simulink model "blank_canvas_ssc"  (R2025b)
settings: Solver=ode1  StartTime=0.0  StopTime=1  FixedStep=Ts  RelTol=1e-3  EnableMultiTasking=on
settings Model: SimulationMode=accelerator  Creator=gdudgeon  LastModifiedBy=gdudgeon
settings SolverCC: AlgebraicLoopSolver=TrustRegion  AutoInsertRateTranBlk=on
settings DataIOCC: ExternalInput=[t, load_inputs]  LoadExternalInput=on  SaveFormat=Array  SaveOutput=off  DSMLogging=off  InspectSignalLogs=on  VisualizeSimOutput=off  SaveTime=off
settings OptimizationCC: ExpressionDepthLimit=2147483647.0  LifeSpan=inf
settings DebuggingCC: UnderspecifiedInitializationDetection=Classic  MergeDetectMultiDrivingBlocksExec=none  SolverPrmCheckMsg=warning  UnconnectedInputMsg=warning  UnconnectedOutputMsg=warning  UnconnectedLineMsg=warning  StateNameClashWarn=warning  SFUnexpectedBacktrackingDiag=warning  SFNoUnconditionalDefaultTransitionDiag=warning  SFExecutionAtInitializationDiag=none  ArithmeticOperatorsInVariantConditions=warning
settings HardwareCC: ProdBitPerPointer=32.0  ProdBitPerSizeT=32.0  ProdBitPerPtrDiffT=32.0  ProdLargestAtomicFloat=None  ProdIntDivRoundTo=Undefined  ProdEndianess=Unspecified  ProdWordSize=32.0  ProdHWDeviceType=32-bit Generic
settings ModelReferenceCC: EnableRefExpFcnMdlSchedulingChecks=on  PropagateSignalLabelsOutOfModel=off
settings SFSimCC: SimUseLocalCustomCode=off  CustomCodeUndefinedFunction=UseInterfaceOnly
settings RTWCC: RTWUseLocalCustomCode=off  GPUComputeCapability=3.5
settings CodeAppCC: StateflowObjectComments=on
settings GRTTargetCC: TargetLangStandard=C89/C90 (ANSI)
settings ConfigComp: CovMetricSettings=dw  CovSaveCumulativeToWorkspaceVar=on  CovSaveSingleToWorkspaceVar=on  CovExternalEMLEnable=off  CovSFcnEnable=off
settings SimscapeCC: SimscapeNormalizeSystem=off
settings ConfigurationSet: Description=SimMechanics 2G

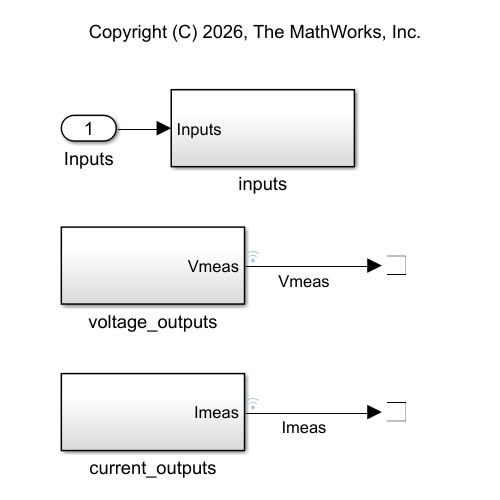
[thumbnail: Simulink's stored preview of the top-level diagram]
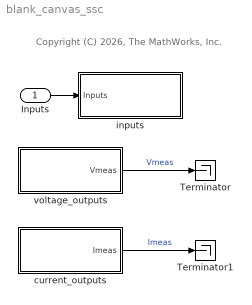
== system blank_canvas_ssc ==
  note: Copyright (C) 2026, The MathWorks, Inc.
  Inputs : Inport
  Terminator : Terminator
  Terminator1 : Terminator
  current_outputs : Subsystem
  inputs : Subsystem
  voltage_outputs : Subsystem
  wires:
  voltage_outputs/1(Vmeas) -> Terminator/1  "Vmeas"
  current_outputs/1(Imeas) -> Terminator1/1  "Imeas"
  Inputs/1 -> inputs/1(Inputs)

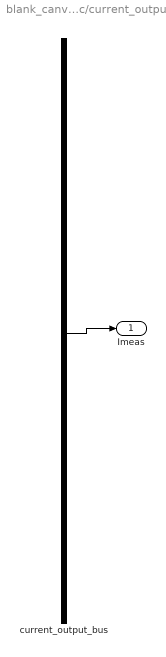
== system blank_canvas_ssc/current_outputs ==
  current_output_bus : BusCreator  Inputs=118
  Imeas : Outport  VectorParamsAs1DForOutWhenUnconnected=off
  wires:
  current_output_bus/1 -> Imeas/1

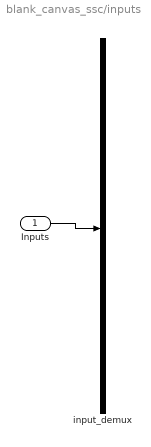
== system blank_canvas_ssc/inputs ==
  Inputs : Inport
  input_demux : Demux  Outputs=76
  wires:
  Inputs/1 -> input_demux/1

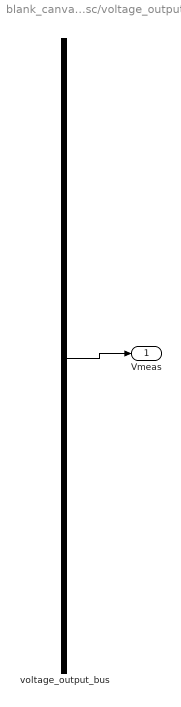
== system blank_canvas_ssc/voltage_outputs ==
  voltage_output_bus : BusCreator  Inputs=128
  Vmeas : Outport  VectorParamsAs1DForOutWhenUnconnected=off
  wires:
  voltage_output_bus/1 -> Vmeas/1
